simulink model "Quadrotor_Model_Y"  (R2016a)
settings: Solver=VariableStepAuto  StartTime=0.0  StopTime=20  RelTol=1e-3
settings Model: Creator=SRQ  LastModifiedBy=SRQ

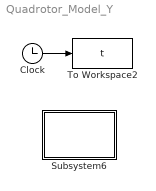
== system Quadrotor_Model_Y ==
  Clock : Clock
  Subsystem6 : Subsystem
      mask Display: disp('Y轴向与翻滚角');
  To Workspace2 : ToWorkspace  VariableName=t  SampleTime=-1
  wires:
  Clock/1 -> To Workspace2/1

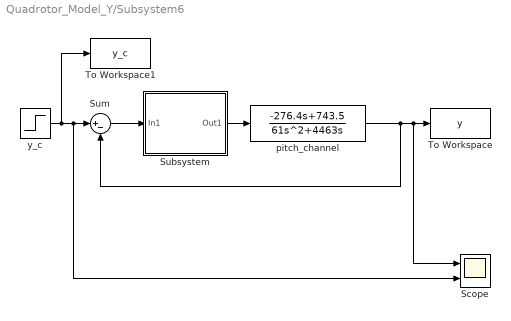
== system Quadrotor_Model_Y/Subsystem6 ==
  Scope : Scope  NumInputPorts=2
  Subsystem : Subsystem  mask{kp=5, ki=0.01, kd=0.1}
      mask Display: disp('PID');
  Sum : Sum  Inputs=|+-
  To Workspace : ToWorkspace  VariableName=y  SampleTime=-1
  To Workspace1 : ToWorkspace  VariableName=y_c  SampleTime=-1
  pitch_channel : TransferFcn  Numerator=[-276.4 743.5]  Denominator=[61 4463 0]
  y_c : Step  Time=0  SampleTime=0
  wires:
  y_c/1 -> To Workspace1/1, Scope/2, Sum/1
  Sum/1 -> Subsystem/1(In1)
  Subsystem/1(Out1) -> pitch_channel/1
  pitch_channel/1 -> Sum/2, Scope/1, To Workspace/1

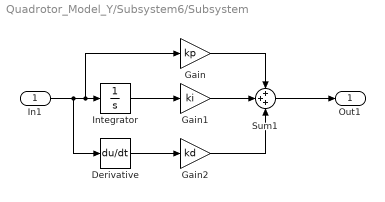
== system Quadrotor_Model_Y/Subsystem6/Subsystem ==
  In1 : Inport
  Derivative : Derivative
  Gain : Gain  Gain=kp
  Gain1 : Gain  Gain=ki
  Gain2 : Gain  Gain=kd
  Integrator : Integrator
  Sum1 : Sum  Inputs=+++
  Out1 : Outport
  wires:
  Integrator/1 -> Gain1/1
  Derivative/1 -> Gain2/1
  Gain2/1 -> Sum1/3
  Gain/1 -> Sum1/1
  In1/1 -> Derivative/1, Gain/1, Integrator/1
  Sum1/1 -> Out1/1
  Gain1/1 -> Sum1/2
